simulink library "control"  (Simulink 7.7)
settings: Solver=ode45  StartTime=0.0  StopTime=10.0  RelTol=1e-3
libraries: simulink x2
settings Model: Creator=corkep  LastModifiedBy=corkep

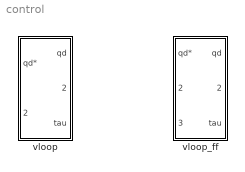
== system control ==
  vloop : Subsystem  mask{J=372e-6, B=817e-6, Km=0.228, tau_max=0.9, Kv=1, Ki=0, T=0.001}
      mask prompts: J "Inertia (J)"; B "Viscous friction coefficient (B)"; Km "Motor torque constant"; tau_max "Torque limit (tau_max)"; Kv "Proportional gain (Kv)"; Ki "Integral gain (Ki)"; T "Sample interval (T)"
  vloop_ff : Subsystem  mask{J=372e-6, B=817e-6, Km=0.228, tau_max=0.9, Kv=1, Ki=0, T=0.001}
      mask prompts: J "Inertia (J)"; B "Viscous friction coefficient (B)"; Km "Motor torque constant"; tau_max "Torque limit (tau_max)"; Kv "Proportional gain (Kv)"; Ki "Integral gain (Ki)"; T "Sample interval (T)"

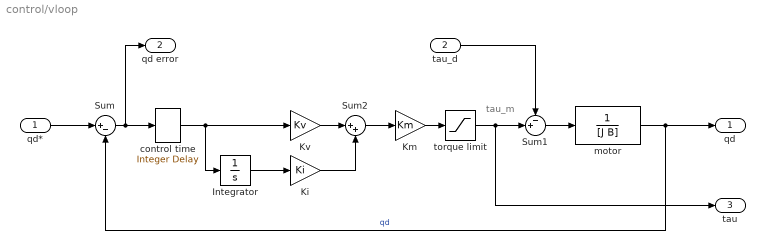
== system control/vloop ==
  note: tau_m
  qd* : Inport
  tau_d : Inport  Port=2
  Integrator : Integrator
  Ki : Gain  Gain=Ki
  Km : Gain  Gain=Km
  Kv : Gain  Gain=Kv
  Sum : Sum  Inputs=|+-
  Sum1 : Sum  Inputs=-+|
  Sum2 : Sum  Inputs=|++
  control time : simulink/Discrete/Integer Delay  NumDelays=1  InputProcessing=Inherited  vinit=0.0  samptime=T
  motor : TransferFcn  Denominator=[J B]  ContinuousStateAttributes='qd'
  torque limit : Saturate  UpperLimit=tau_max  LowerLimit=-tau_max
  qd : Outport
  qd error : Outport  Port=2
  tau : Outport  Port=3
  wires:
  Ki/1 -> Sum2/2
  Integrator/1 -> Ki/1
  Kv/1 -> Sum2/1
  Sum2/1 -> Km/1
  Km/1 -> torque limit/1
  qd*/1 -> Sum/1
  control time/1 -> Integrator/1, Kv/1
  torque limit/1 -> tau/1, Sum1/2
  tau_d/1 -> Sum1/1
  motor/1 -> qd/1, Sum/2  "qd"
  Sum/1 -> qd error/1, control time/1
  Sum1/1 -> motor/1

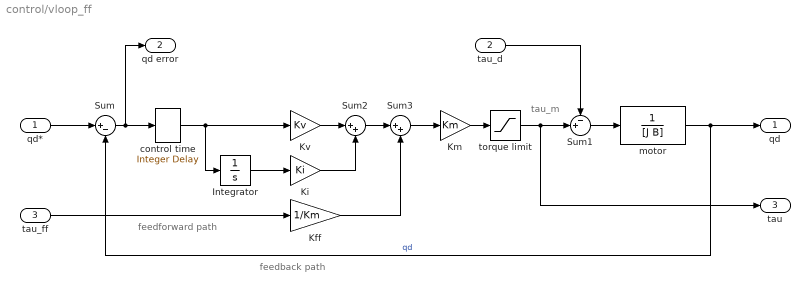
== system control/vloop_ff ==
  note: tau_m
  note: feedforward path
  note: feedback path
  qd* : Inport
  tau_d : Inport  Port=2
  tau_ff : Inport  Port=3
  Integrator : Integrator
  Kff : Gain  Gain=1/Km
  Ki : Gain  Gain=Ki
  Km : Gain  Gain=Km
  Kv : Gain  Gain=Kv
  Sum : Sum  Inputs=|+-
  Sum1 : Sum  Inputs=-+|
  Sum2 : Sum  Inputs=|++
  Sum3 : Sum  Inputs=|++
  control time : simulink/Discrete/Integer Delay  NumDelays=1  InputProcessing=Inherited  vinit=0.0  samptime=T
  motor : TransferFcn  Denominator=[J B]  ContinuousStateAttributes='qd'
  torque limit : Saturate  UpperLimit=tau_max  LowerLimit=-tau_max
  qd : Outport
  qd error : Outport  Port=2
  tau : Outport  Port=3
  wires:
  Sum1/1 -> motor/1
  Sum/1 -> control time/1, qd error/1
  motor/1 -> qd/1, Sum/2  "qd"
  tau_d/1 -> Sum1/1
  torque limit/1 -> Sum1/2, tau/1
  control time/1 -> Kv/1, Integrator/1
  qd*/1 -> Sum/1
  Km/1 -> torque limit/1
  Kv/1 -> Sum2/1
  Integrator/1 -> Ki/1
  Ki/1 -> Sum2/2
  Sum2/1 -> Sum3/1
  Sum3/1 -> Km/1
  Kff/1 -> Sum3/2
  tau_ff/1 -> Kff/1
